simulink model "MPSLab3"  (R2014b)
settings: Solver=ode3  StartTime=0.0  StopTime=20.0  FixedStep=0.01  RelTol=1e-3
undefined symbols (not defined in the file): magnitude
settings Model: Creator=kiril_000  LastModifiedBy=kiril_000

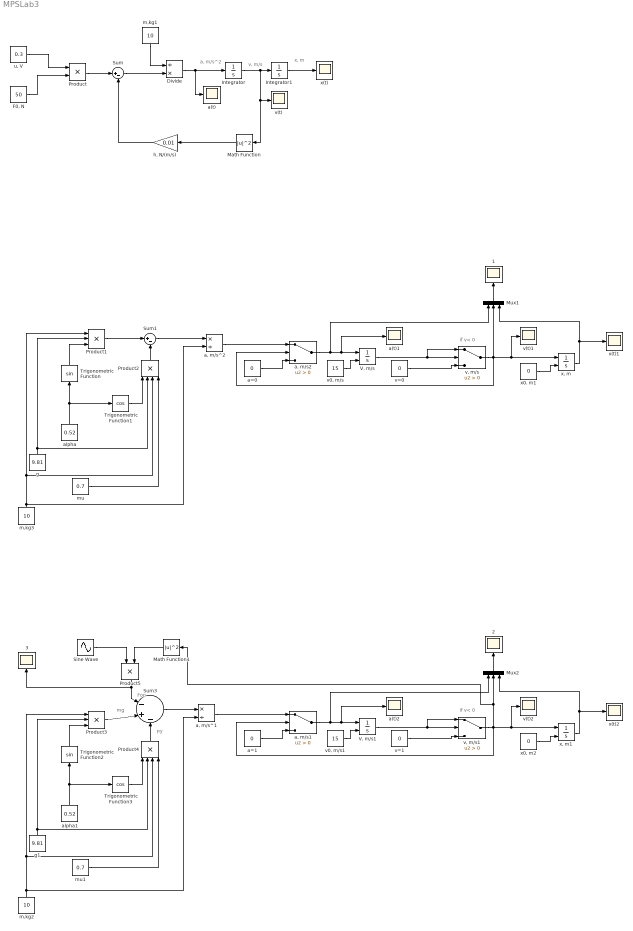
== system MPSLab3 ==
  note: Fop
  note: Ftr
  note: mg
  note: if v< 0
  note: x, m
  note: v, m/s
  note: a, m/s^2
  note: if v< 0
  "  1" : Scope
      settings: ShowLegends=on  TimeRange=65  YMin=-10  YMax=70  SaveName=ScopeData10
  "  2" : Scope
      settings: ShowLegends=on  TimeRange=65  YMin=-10  YMax=70  SaveName=ScopeData6
  "  3" : Scope
      settings: ShowLegends=on  TimeRange=65  YMin=-10  YMax=70  SaveName=ScopeData11
  " v(t)" : Scope
      settings: SaveName=ScopeData2
  " v(t)1" : Scope
      settings: SaveName=ScopeData3
  " v(t)2" : Scope
      settings: SaveName=ScopeData7
  Divide : Product  Inputs=/*
  "F0, N" : Constant  Value=50
  Integrator : Integrator
  Integrator1 : Integrator
  Math Function : Math  Operator=magnitude^2  SaturateOnIntegerOverflow=on
  Math Function1 : Math  Operator=magnitude^2  SaturateOnIntegerOverflow=on
  Mux1 : Mux  Inputs=3
  Mux2 : Mux  Inputs=3
  Product : Product
  Product1 : Product  Inputs=3
  Product2 : Product  Inputs=4
  Product3 : Product  Inputs=3
  Product4 : Product  Inputs=4
  Product5 : Product
  Sine Wave : Sin  Amplitude=0.001  Frequency=10  SampleTime=0
  Sum : Sum  Inputs=|+-
  Sum1 : Sum  Inputs=|+-
  Sum3 : Sum  Inputs=|-+-
  Trigonometric Function : Trigonometry  ApproximationMethod=CORDIC
  Trigonometric Function1 : Trigonometry  Operator=cos  ApproximationMethod=CORDIC
  Trigonometric Function2 : Trigonometry  ApproximationMethod=CORDIC
  Trigonometric Function3 : Trigonometry  Operator=cos  ApproximationMethod=CORDIC
  "V, m/s" : Integrator  InitialConditionSource=external
  "V, m/s1" : Integrator  InitialConditionSource=external
  a(t) : Scope
  a(t)1 : Scope
      settings: YMin=-1.5  YMax=1  SaveName=ScopeData4
  a(t)2 : Scope
      settings: YMin=-1.5  YMax=1  SaveName=ScopeData8
  "a, m/s1" : Switch  Criteria=u2 > Threshold
  "a, m/s2" : Switch  Criteria=u2 > Threshold
  "a, m/s^1" : Product  Inputs=*/
  "a, m/s^2" : Product  Inputs=*/
  a=0 : Constant  Value=0
  a=1 : Constant  Value=0
  alpha : Constant  Value=0.52
  alpha1 : Constant  Value=0.52
  g : Constant  Value=9.81
  g1 : Constant  Value=9.81
  "h, N/(m/s)" : Gain  Gain=0.01
  m,kg1 : Constant  Value=10
  m,kg2 : Constant  Value=10
  m,kg3 : Constant  Value=10
  mu : Constant  Value=0.7
  mu1 : Constant  Value=0.7
  "u, V " : Constant  Value=0.3
  "v, m/s" : Switch  Criteria=u2 > Threshold
  "v, m/s1" : Switch  Criteria=u2 > Threshold
  "v0, m/s" : Constant  Value=15
  "v0, m/s1" : Constant  Value=15
  v=0 : Constant  Value=0
  v=1 : Constant  Value=0
  x(t) : Scope
  x(t)1 : Scope
      settings: TimeRange=10  YMin=799  YMax=801  SaveName=ScopeData5
  x(t)2 : Scope
      settings: TimeRange=10  YMin=799  YMax=801  SaveName=ScopeData9
  "x, m" : Integrator  InitialConditionSource=external
  "x, m1" : Integrator  InitialConditionSource=external
  "x0, m1" : Constant  Value=0
  "x0, m2" : Constant  Value=0
  wires:
  "u, V "/1 -> Product/1
  "F0, N"/1 -> Product/2
  Product/1 -> Sum/1
  Sum/1 -> Divide/2
  m,kg1/1 -> Divide/1
  Divide/1 -> a(t)/1, Integrator/1
  Integrator/1 -> Math Function/1, " v(t)"/1, Integrator1/1
  Integrator1/1 -> x(t)/1
  Math Function/1 -> "h, N/(m/s)"/1
  "h, N/(m/s)"/1 -> Sum/2
  g/1 -> Product2/2, Product1/2
  alpha/1 -> Trigonometric Function/1, Trigonometric Function1/1
  Trigonometric Function/1 -> Product1/3
  Product1/1 -> Sum1/1
  Product2/1 -> Sum1/2
  Trigonometric Function1/1 -> Product2/1
  mu/1 -> Product2/4
  "x, m"/1 -> x(t)1/1, Mux1/3
  "v0, m/s"/1 -> "V, m/s"/2
  "x0, m1"/1 -> "x, m"/2
  Sine Wave/1 -> Product5/1
  Math Function1/1 -> Product5/2
  Sum1/1 -> "a, m/s^2"/1
  v=0/1 -> "v, m/s"/3
  "V, m/s"/1 -> "v, m/s"/1, "v, m/s"/2
  "v, m/s"/1 -> Mux1/2, "x, m"/1, " v(t)1"/1, "a, m/s2"/2
  Mux1/1 -> "  1"/1
  m,kg2/1 -> "a, m/s^1"/2, Product3/1, Product4/3
  g1/1 -> Product3/2, Product4/2
  alpha1/1 -> Trigonometric Function3/1, Trigonometric Function2/1
  Trigonometric Function2/1 -> Product3/3
  Trigonometric Function3/1 -> Product4/1
  mu1/1 -> Product4/4
  Product3/1 -> Sum3/2
  Product4/1 -> Sum3/3
  Product5/1 -> "  3"/1, Sum3/1
  Sum3/1 -> "a, m/s^1"/1
  m,kg3/1 -> Product2/3, Product1/1, "a, m/s^2"/2
  a=0/1 -> "a, m/s2"/3
  "a, m/s^2"/1 -> "a, m/s2"/1
  "a, m/s2"/1 -> Mux1/1, a(t)1/1, "V, m/s"/1
  "x, m1"/1 -> x(t)2/1, Mux2/3
  "v0, m/s1"/1 -> "V, m/s1"/2
  "x0, m2"/1 -> "x, m1"/2
  v=1/1 -> "v, m/s1"/3
  "V, m/s1"/1 -> "v, m/s1"/1, "v, m/s1"/2
  "v, m/s1"/1 -> Math Function1/1, Mux2/2, "x, m1"/1, " v(t)2"/1, "a, m/s1"/2
  Mux2/1 -> "  2"/1
  a=1/1 -> "a, m/s1"/3
  "a, m/s^1"/1 -> "a, m/s1"/1
  "a, m/s1"/1 -> Mux2/1, a(t)2/1, "V, m/s1"/1
